simulink model "DAB"  (R2020a)
settings: Solver=VariableStepAuto  StartTime=0.0  StopTime=1  RelTol=1e-3
libraries: powerlib x15
settings Model: Creator=Matthew  LastModifiedBy=Matthew

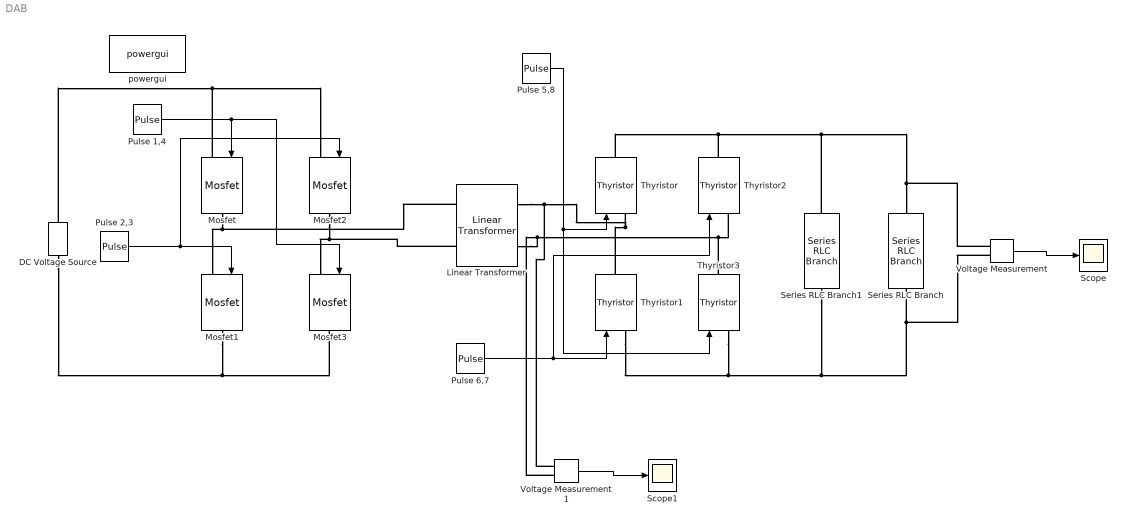
== system DAB ==
  DC Voltage Source : powerlib/Electrical Sources/DC Voltage Source  Amplitude=100  Measurements=None
  Linear Transformer : powerlib/Elements/Linear Transformer  UNITS=SI  NominalPower=[ 20000 10000 ]  winding1=[500 4.3218 0.45856]  winding2=[250 0.7938 0.084225]  ThreeWindings=off  winding3=[3.15e+05 0.7938 0.084225]  RmLm=[1.0805e+06 2866]  Measurements=None  DataType=on
  Mosfet{,1..3} (4 alike) : powerlib/Power Electronics/Mosfet  Ron=0.1  Lon=0  Rd=0.01  Vfd=0  IC=0  Rs=1e5  Cs=inf  Measurements=off
  Pulse 1,4 : DiscretePulseGenerator  PulseType=Time based  Amplitude=10  Period=100e-6  PulseWidth=50
  Pulse 2,3 : DiscretePulseGenerator  PulseType=Time based  Amplitude=10  Period=100e-6  PulseWidth=50  PhaseDelay=50e-6
  Pulse 5,8 : DiscretePulseGenerator  PulseType=Time based  Amplitude=10  Period=100e-6  PulseWidth=50
  Pulse 6,7 : DiscretePulseGenerator  PulseType=Time based  Amplitude=10  Period=100e-6  PulseWidth=50  PhaseDelay=50e-6
  Scope : Scope
  Scope1 : Scope
  Series RLC Branch : powerlib/Elements/Series RLC Branch  LConnTagsString=__new0  RConnTagsString=__new0  BranchType=R  Resistance=1  Inductance=1e-3  SetiL0=off  InitialCurrent=0  Capacitance=1e-6  Setx0=off  InitialVoltage=0  Measurements=None
  Series RLC Branch1 : powerlib/Elements/Series RLC Branch  LConnTagsString=__new0  RConnTagsString=__new0  BranchType=C  Resistance=1  Inductance=1e-3  SetiL0=off  InitialCurrent=0  Capacitance=1e-6  Setx0=off  InitialVoltage=0  Measurements=None
  Thyristor{,1..3} (4 alike) : powerlib/Power Electronics/Thyristor  Ron=0.001  Lon=0  Vf=0.8  IC=0  Rs=500  Cs=250e-9  Measurements=off
  Voltage Measurement : powerlib/Measurements/Voltage Measurement  PhasorSimulation=off  OutputType=Complex  PSBequivalent=0
  Voltage Measurement1 : powerlib/Measurements/Voltage Measurement  PhasorSimulation=off  OutputType=Complex  PSBequivalent=0
  powergui : powerlib/powergui  Priority=1  SimulationMode=Continuous  SampleTime=50e-6  frequency=60  Iterations=50  frequencyindice=0  Pbase=100e6  ErrMax=1e-4  UnitsV=kV  UnitsW=MW  buscounter=0  FunctionMessages=off  echomessages=off  EnableUseOfTLC=off  CurrentSourceSwitches=off  DisableSnubberDevices=off  DisableRonSwitches=off  DisableVfSwitches=off  DisplayEquations=off  AutomaticDiscreteSolvers=off  SolverType=Tustin/Backward Euler (TBE)  Interpol=off  ExternalGateDelay=off  methode=off  Ts=100  x0status=blocks  SPID=on  SwTol=0  HookPort=off  NonlinearTolerance=1e-4  nMaxIteration=100  ContinueOnMaxIteration=off  RestoreLinks=warning  ResistiveCurrentMeasurement=off  Frange=[0:2:500]  Ylog=off  Xlog=on  ShowGrid=off  save=off  variable=ZData  structure=0  ZoomFFT=off  StartTime=0.0  cycles=1  DisplayStyle=1  fundamental=60  FreqAxis=off  MaxFrequency=1000  frequencyindicesteady=1  RmsSteady=1  display=off
  wires:
  Pulse 2,3/1 -> Mosfet2/1, Mosfet1/1
  Pulse 1,4/1 -> Mosfet3/1, Mosfet/1
  Voltage Measurement/1 -> Scope/1
  Pulse 5,8/1 -> Thyristor3/1, Thyristor/1
  Pulse 6,7/1 -> Thyristor2/1, Thyristor1/1
  Voltage Measurement1/1 -> Scope1/1
  connections:
  Mosfet/RConn1 -- Mosfet1/LConn1 -- Linear Transformer/LConn1
  Mosfet2/RConn1 -- Mosfet3/LConn1 -- Linear Transformer/LConn2
  Thyristor1/RConn1 -- Voltage Measurement1/LConn1 -- Linear Transformer/RConn1 -- Thyristor/LConn1
  Thyristor3/RConn1 -- Thyristor2/LConn1 -- Voltage Measurement1/LConn2 -- Linear Transformer/RConn2
  DC Voltage Source/RConn1 -- Mosfet/LConn1 -- Mosfet2/LConn1
  DC Voltage Source/LConn1 -- Mosfet1/RConn1 -- Mosfet3/RConn1
  Thyristor/RConn1 -- Series RLC Branch1/LConn1 -- Voltage Measurement/LConn1 -- Series RLC Branch/LConn1 -- Thyristor2/RConn1
  Thyristor1/LConn1 -- Thyristor3/LConn1 -- Series RLC Branch1/RConn1 -- Voltage Measurement/LConn2 -- Series RLC Branch/RConn1
